simulink model "aprbs"  (Simulink 7.3)
settings: Solver=ode45  StartTime=0.0  StopTime=100.0  RelTol=1e-3
settings Model: Creator=Daniel  LastModifiedBy=Daniel

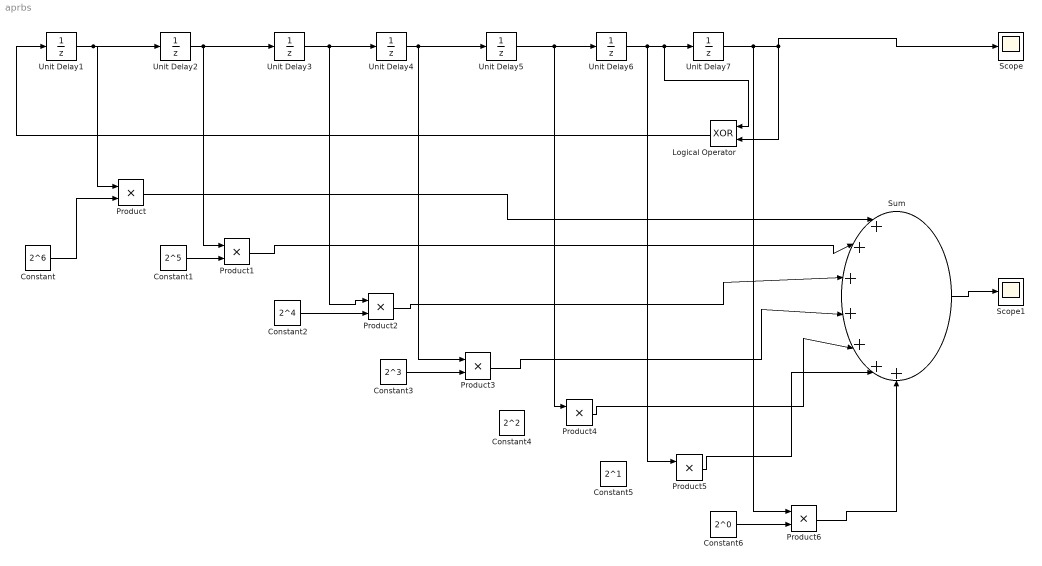
== system aprbs ==
  Constant : Constant  Value=2^6  OutDataType=fixdt(1, 16)  OutScaling=2^0
  Constant1 : Constant  Value=2^5  OutDataType=fixdt(1, 16)  OutScaling=2^0
  Constant2 : Constant  Value=2^4  OutDataType=fixdt(1, 16)  OutScaling=2^0
  Constant3 : Constant  Value=2^3  OutDataType=fixdt(1, 16)  OutScaling=2^0
  Constant4 : Constant  Value=2^2  OutDataType=fixdt(1, 16)  OutScaling=2^0
  Constant5 : Constant  Value=2^1  OutDataType=fixdt(1, 16)  OutScaling=2^0
  Constant6 : Constant  Value=2^0  OutDataType=fixdt(1, 16)  OutScaling=2^0
  Logical Operator : Logic  Operator=XOR  AllPortsSameDT=off  OutDataTypeMode=boolean  LogicDataType=fixdt(0, 8)  OutDataTypeStr=boolean
  Product{,1..6} (7 alike) : Product  OutDataType=fixdt(1, 16)  OutScaling=2^0  RndMeth=Zero
  Scope : Scope
      settings: DataFormat=Array
  Scope1 : Scope
  Sum : Sum  Inputs=|+++++++  OutDataType=fixdt(1, 16)  OutScaling=2^0
  Unit Delay{1..7} (7 alike) : UnitDelay  X0=1
  wires:
  Unit Delay1/1 -> Unit Delay2/1, Product/1
  Unit Delay2/1 -> Unit Delay3/1, Product1/1
  Unit Delay3/1 -> Unit Delay4/1, Product2/1
  Unit Delay4/1 -> Unit Delay5/1, Product3/1
  Unit Delay5/1 -> Unit Delay6/1, Product4/1
  Logical Operator/1 -> Unit Delay1/1
  Unit Delay6/1 -> Unit Delay7/1, Logical Operator/1, Product5/1
  Unit Delay7/1 -> Logical Operator/2, Scope/1, Product6/1
  Product/1 -> Sum/1
  Product1/1 -> Sum/2
  Product2/1 -> Sum/3
  Product3/1 -> Sum/4
  Product4/1 -> Sum/5
  Product5/1 -> Sum/6
  Product6/1 -> Sum/7
  Constant/1 -> Product/2
  Constant1/1 -> Product1/2
  Constant2/1 -> Product2/2
  Constant3/1 -> Product3/2
  Constant6/1 -> Product6/2
  Sum/1 -> Scope1/1
